simulink model "RC_K10"  (R2025a)
settings: Solver=VariableStepAuto  StartTime=0.0  StopTime=500e-6  MaxStep=5.3e-6/25  RelTol=1e-3
libraries: MK_K x3
settings Model: Creator=Szalay  LastModifiedBy=Szalay

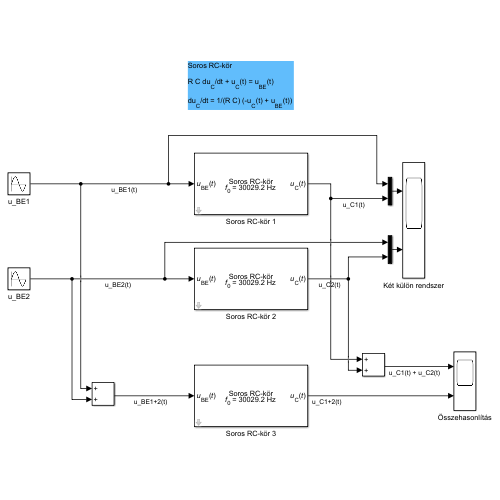
[thumbnail: Simulink's stored preview of the top-level diagram]
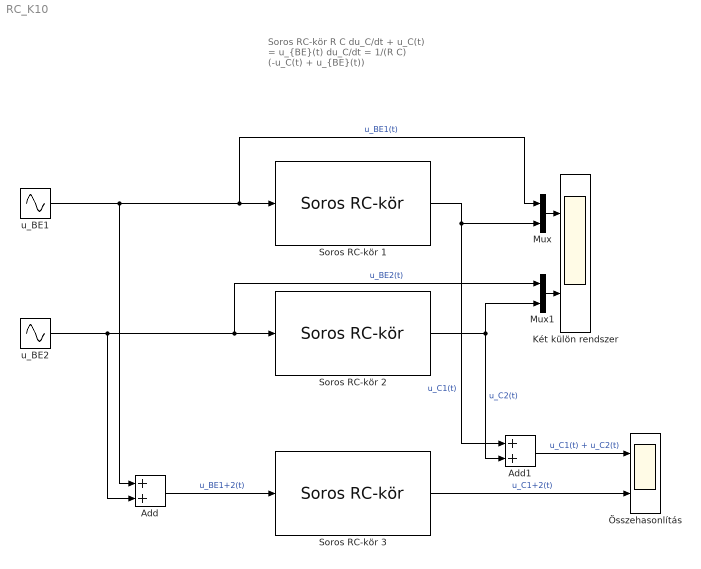
== system RC_K10 ==
  note: Soros RC-kör
      |
      | R C du_C/dt + u_C(t) = u_{BE}(t)
      |
      | du_C/dt = 1/(R C) (-u_C(t) + u_{BE}(t))
  Add : Sum
  Add1 : Sum
  Két külön rendszer : Scope  NumInputPorts=2
      settings: ActiveDisplayYMinimum=-1.25  ActiveDisplayYMaximum=1.25
  Mux : Mux  Inputs=2
  Mux1 : Mux  Inputs=2
  Soros RC-kör 1 : MK_K/Soros RC-kör  R=1  C=5.3e-6  u_C0=0
  Soros RC-kör 2 : MK_K/Soros RC-kör  R=1  C=5.3e-6  u_C0=0
  Soros RC-kör 3 : MK_K/Soros RC-kör  R=1  C=5.3e-6  u_C0=0
  u_BE1 : Sin  Frequency=2*pi*10000  SampleTime=0
  u_BE2 : Sin  Frequency=2*pi*100000  SampleTime=0
  Összehasonlítás : Scope  NumInputPorts=2
      settings: ActiveDisplayYMinimum=-1.5404719246060974  ActiveDisplayYMaximum=1.5066075398333665
  wires:
  u_BE2/1 -> Add/2, Mux1/1, Soros RC-kör 2/1  "u_BE2(t)"
  u_BE1/1 -> Add/1, Mux/1, Soros RC-kör 1/1  "u_BE1(t)"
  Soros RC-kör 1/1 -> Mux/2, Add1/1  "u_C1(t)"
  Soros RC-kör 2/1 -> Mux1/2, Add1/2  "u_C2(t)"
  Mux/1 -> Két külön rendszer/1
  Mux1/1 -> Két külön rendszer/2
  Add/1 -> Soros RC-kör 3/1  "u_BE1+2(t)"
  Soros RC-kör 3/1 -> Összehasonlítás/2  "u_C1+2(t)"
  Add1/1 -> Összehasonlítás/1  "u_C1(t) + u_C2(t)"
